simulink model "Heating_Two_Rooms_Kalman"  (R2022b)
settings: Solver=VariableStepAuto  StartTime=0.0  StopTime=3600.0  RelTol=1e-3
values from neighbouring files (symbols this model uses):
  A = [-(h*A_s+k)/C1, k/C1 ... (first row only)    [TwoRooms.m]
  B = [1/C1 0; 0, 1/C2]    [TwoRooms.m]
  C = [1 0; 0 1]    [TwoRooms.m]
  D = 0*eye(2)    [TwoRooms.m]
  R = 100*eye(2)    [TwoRooms.m]
undefined symbols (not defined in the file or in its folder): Continuous, K1, Time
libraries: simulink x2, ctrlSharedLib x1
settings Model: Creator=logan  LastModifiedBy=oluwafemiajeigbe

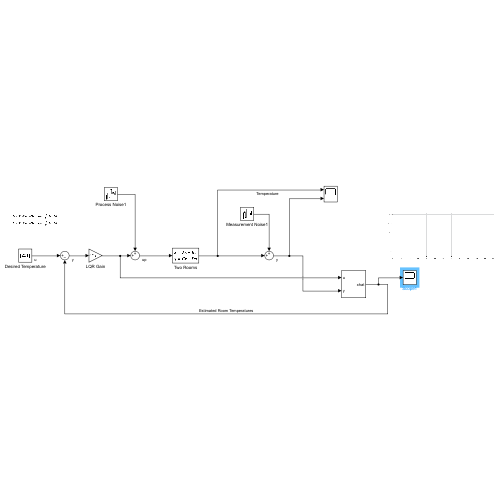
[thumbnail: Simulink's stored preview of the top-level diagram]
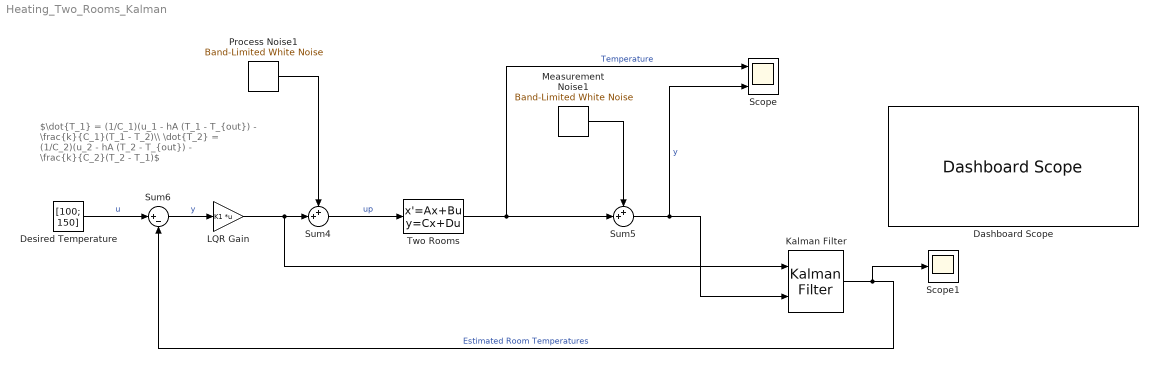
== system Heating_Two_Rooms_Kalman ==
  note: $\dot{T_1} = (1/C_1)(u_1 - hA (T_1 - T_{out}) - \frac{k}{C_1}(T_1 - T_2)\\ \dot{T_2} = (1/C_2)(u_2 - hA (T_2 - T_{out}) - \frac{k}{C_2}(T_2 - T_1)$
  Dashboard Scope : DashboardScope
  Desired Temperature : Constant  Value=[100; 150]
  Kalman Filter : ctrlSharedLib/Kalman Filter  TimeDomain=Continuous-Time  UseCurrentEstimator=on  ModelSource=Individual A, B, C, D matrices  ModelSourceVariable=Plant  A=A  B=B  C=C  D=D  NumberOfStates=1  NumberOfInputs=1  NumberOfOutputs=1  InitialEstimateSource=Dialog  X0=20  P0=10  UseK=off  UseGH=on  NumberOfProcessNoiseInputs=1  G=G  TimeInvariantG=on  H=0  TimeInvariantH=on  Q=Q  TimeInvariantQ=on  R=R  TimeInvariantR=on  N=0  TimeInvariantN=on  AddInputPort=on  AddEnablePort=off  OutputEstimatedY=off  OutputP=off  Ts=-1
  LQR Gain : Gain  Gain=K1  Multiplication=Matrix(K*u)
  Measurement Noise1 : simulink/Sources/Band-Limited White Noise  Cov=[0.1 0.1]  Ts=0.1  seed=[23341]
  Process Noise1 : simulink/Sources/Band-Limited White Noise  Cov=[0.1]  Ts=0.1  seed=[23341]
  Scope : Scope  NumInputPorts=2
  Scope1 : Scope
  Sum4 : Sum  Inputs=++|
  Sum5 : Sum  Inputs=++|
  Sum6 : Sum  Inputs=|+-
  Two Rooms : StateSpace  A=A  B=B  C=C  D=D  InitialCondition=20
  wires:
  Kalman Filter/1 -> Scope1/1, Sum6/2  "Estimated Room Temperatures"
  Desired Temperature/1 -> Sum6/1  "u"
  Sum6/1 -> LQR Gain/1  "y"
  LQR Gain/1 -> Kalman Filter/1, Sum4/2
  Process Noise1/1 -> Sum4/1
  Sum4/1 -> Two Rooms/1  "up"
  Two Rooms/1 -> Scope/1, Sum5/2  "Temperature"
  Sum5/1 -> Scope/2, Kalman Filter/2  "y"
  Measurement Noise1/1 -> Sum5/1
